simulink model "fuzzyModel"  (R2017a)
settings: Solver=VariableStepAuto  StartTime=0.0  StopTime=500.0  RelTol=1e-3
values from neighbouring files (symbols this model uses):
  den = [1 5 6.75 2.25]    [main.m]
  num = 2    [main.m]
  timeDelay = minRoot/3    [main.m]
libraries: fuzblock x4
settings Model: Creator=jpleitao  LastModifiedBy=jpleitao

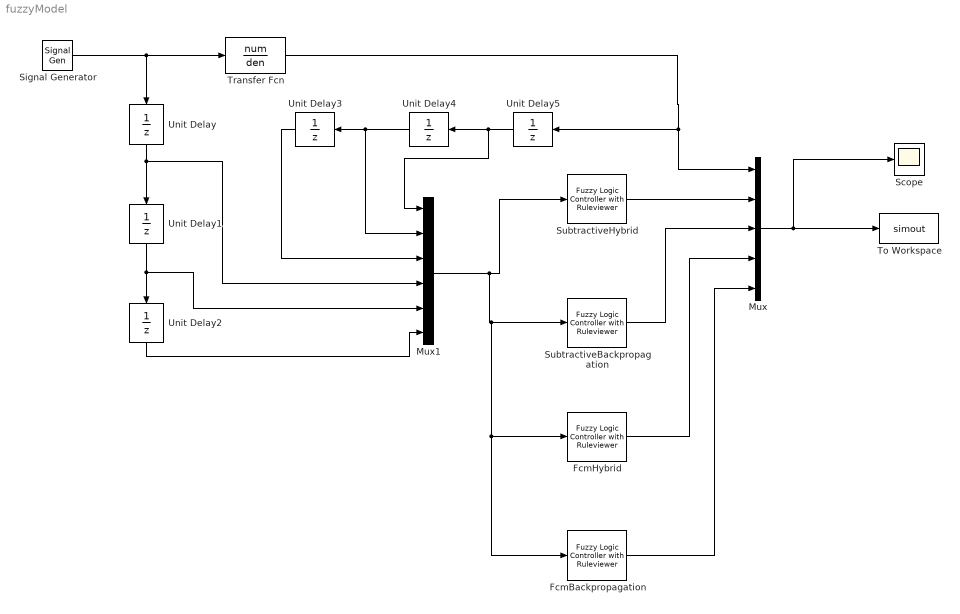
== system fuzzyModel ==
  FcmBackpropagation : fuzblock/Fuzzy Logic  Controller  with Ruleviewer  fismatrix=fcmBackAnfis  Ts=timeDelay
  FcmHybrid : fuzblock/Fuzzy Logic  Controller  with Ruleviewer  fismatrix=fcmHybridAnfis  Ts=timeDelay
  Mux : Mux  Inputs=5
  Mux1 : Mux  Inputs=6
  Scope : Scope
  Signal Generator : SignalGenerator  WaveForm=sawtooth  Frequency=timeDelay
  SubtractiveBackpropagation : fuzblock/Fuzzy Logic  Controller  with Ruleviewer  fismatrix=subtractiveBackAnfis  Ts=timeDelay
  SubtractiveHybrid : fuzblock/Fuzzy Logic  Controller  with Ruleviewer  fismatrix=subtractiveHybridAnfis  Ts=timeDelay
  To Workspace : ToWorkspace  VariableName=simout  SaveFormat=Structure With Time  SampleTime=timeDelay
  Transfer Fcn : TransferFcn  Numerator=num  Denominator=den
  Unit Delay{,1..5} (6 alike) : UnitDelay  SampleTime=timeDelay
  wires:
  Signal Generator/1 -> Unit Delay/1, Transfer Fcn/1
  Unit Delay1/1 -> Mux1/5, Unit Delay2/1
  Transfer Fcn/1 -> Unit Delay5/1, Mux/1
  Mux/1 -> To Workspace/1, Scope/1
  Unit Delay5/1 -> Mux1/1, Unit Delay4/1
  Unit Delay3/1 -> Mux1/3
  Unit Delay4/1 -> Mux1/2, Unit Delay3/1
  Unit Delay/1 -> Mux1/4, Unit Delay1/1
  Unit Delay2/1 -> Mux1/6
  Mux1/1 -> FcmBackpropagation/1, FcmHybrid/1, SubtractiveBackpropagation/1, SubtractiveHybrid/1
  SubtractiveHybrid/1 -> Mux/2
  SubtractiveBackpropagation/1 -> Mux/3
  FcmHybrid/1 -> Mux/4
  FcmBackpropagation/1 -> Mux/5
